simulink model "testDeriv"  (R2018b)
settings: Solver=FixedStepAuto  StartTime=0.0  StopTime=30  FixedStep=0.0125  RelTol=1e-3
libraries: simulink x3
settings Model: Creator=barthal  LastModifiedBy=barthal

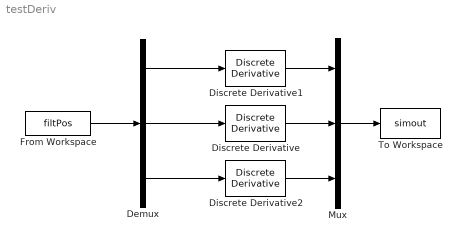
== system testDeriv ==
  Demux : Demux  Outputs=3
  Discrete Derivative : simulink/Discrete/Discrete Derivative  gainval=1.0  ICPrevScaledInput=0.0  InputProcessing=Columns as channels (frame based)  OutMin=[]  OutMax=[]  OutDataType=fixdt(1, 16)  OutScaling=2^-10  DoSatur=off
  Discrete Derivative1 : simulink/Discrete/Discrete Derivative  gainval=1.0  ICPrevScaledInput=0.0  InputProcessing=Columns as channels (frame based)  OutMin=[]  OutMax=[]  OutDataType=fixdt(1, 16)  OutScaling=2^-10  DoSatur=off
  Discrete Derivative2 : simulink/Discrete/Discrete Derivative  gainval=1.0  ICPrevScaledInput=0.0  InputProcessing=Columns as channels (frame based)  OutMin=[]  OutMax=[]  OutDataType=fixdt(1, 16)  OutScaling=2^-10  DoSatur=off
  From Workspace : FromWorkspace  VariableName=filtPos  SampleTime=0
  Mux : Mux  Inputs=3
  To Workspace : ToWorkspace  VariableName=simout  SaveFormat=Timeseries  SampleTime=-1
  wires:
  From Workspace/1 -> Demux/1
  Demux/2 -> Discrete Derivative/1
  Demux/3 -> Discrete Derivative2/1
  Demux/1 -> Discrete Derivative1/1
  Discrete Derivative1/1 -> Mux/1
  Discrete Derivative/1 -> Mux/2
  Discrete Derivative2/1 -> Mux/3
  Mux/1 -> To Workspace/1
